simulink model "c8mchaos_v"  (R2019b)
settings: Solver=ode15s  StartTime=0.0  StopTime=500  RelTol=1e-9  EnableMultiTasking=on
PreLoadFcn:
  | alpha=[0.93,0.99,0.92]; x0=[0.2; -0.1; 0.1];
  | ww=[1e-4 1e3]; N=13;
undefined symbols (not defined in the file): G
libraries: cstblocks x3
settings Model: Creator=Dingyu  LastModifiedBy=xuedi
settings DataIOCC: SaveFormat=Array  ReturnWorkspaceOutputs=off
settings OptimizationCC: LifeSpan=inf
settings DebuggingCC: SFUnexpectedBacktrackingDiag=warning  SFNoUnconditionalDefaultTransitionDiag=warning  ArithmeticOperatorsInVariantConditions=warning
settings SFSimCC: SimUseLocalCustomCode=off  CustomCodeUndefinedFunction=UseInterfaceOnly
settings RTWCC: RTWUseLocalCustomCode=off
settings CodeAppCC: StateflowObjectComments=on
settings GRTTargetCC: TargetLangStandard=C89/C90 (ANSI)
settings ConfigComp: CovMetricSettings=dw  CovSaveCumulativeToWorkspaceVar=on  CovSaveSingleToWorkspaceVar=on  CovExternalEMLEnable=off

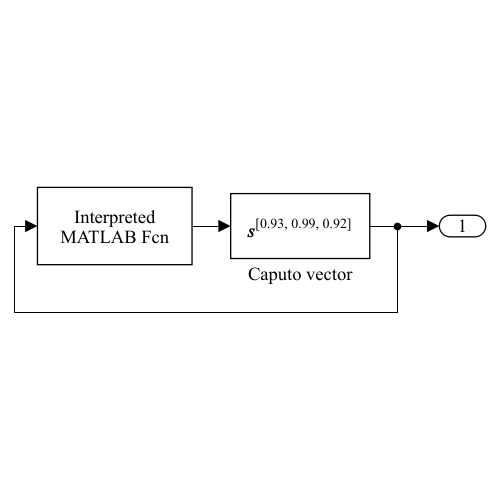
[thumbnail: Simulink's stored preview of the top-level diagram]
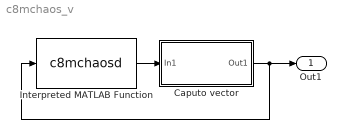
== system c8mchaos_v ==
  Caputo vector : Subsystem  mask{gam=alpha, ww=ww, N=N, M=3, x0=x0}
      mask prompts: gam "Derivative order gamma"; ww "Frequency range [wb,wh]"; N "Apprixmation order N"; M "Dimension M"; x0 "Initial condition x0"
      mask init:
      | wb=ww(1); wh=ww(2); stri=[];
      |    if length(gam)==1, gam=gam*ones(M,1); end
      |    for i=1:M
      |        G(i,1)=ousta_fod(1-gam(i),N,wb,wh); stri=[stri,num2str(gam(i)),', '];
      |    end
      |    str=['{\bf{\its}}^{[' stri(1:end-2) ']}'];
      |    svec2sl(gam);
      mask Display: disp(str,'texmode','on')
  Interpreted MATLAB Function : MATLABFcn  MATLABFcn=c8mchaosd
  Out1 : Outport
  wires:
  Interpreted MATLAB Function/1 -> Caputo vector/1(In1)
  Caputo vector/1(Out1) -> Out1/1, Interpreted MATLAB Function/1

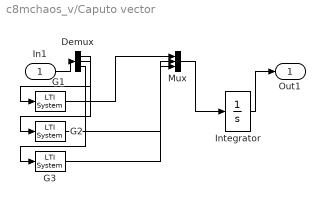
== system c8mchaos_v/Caputo vector ==
  In1 : Inport
  Demux : Demux  Outputs=3
  G1 : cstblocks/LTI System  sys=G(1)  IC=[]
  G2 : cstblocks/LTI System  sys=G(2)  IC=[]
  G3 : cstblocks/LTI System  sys=G(3)  IC=[]
  Integrator : Integrator  InitialCondition=x0
  Mux : Mux  Inputs=3
  Out1 : Outport
  wires:
  Demux/1 -> G1/1
  G1/1 -> Mux/1
  Demux/2 -> G2/1
  G2/1 -> Mux/2
  Demux/3 -> G3/1
  G3/1 -> Mux/3
  Integrator/1 -> Out1/1
  Mux/1 -> Integrator/1
  In1/1 -> Demux/1
